simulink model "MLC_IPC_ctrl_r2018a"  (R2018a)
settings: Solver=ode4  StartTime=0.0  StopTime=Parameter.Time.TMax  FixedStep=Parameter.Time.dt  RelTol=1e-3  EnableMultiTasking=on
undefined symbols (not defined in the file or in its folder): Parameter, x2_t0
libraries: simulink x4
settings Model: Creator=Phoenix_Shao  LastModifiedBy=thisi
settings DataIOCC: MaxDataPoints=1000000  SaveFormat=Array  DSMLogging=off
settings OptimizationCC: ExpressionDepthLimit=2147483647  InitFltsAndDblsToZero=on  EfficientMapNaN2IntZero=off  LifeSpan=inf
settings DebuggingCC: SaveWithParameterizedLinksMsg=none  UnderspecifiedInitializationDetection=Classic  MergeDetectMultiDrivingBlocksExec=none  SignalResolutionControl=TryResolveAllWithWarning  SolverPrmCheckMsg=warning  MultiTaskDSMMsg=warning  MultiTaskCondExecSysMsg=none  FcnCallInpInsideContextMsg=warning  AllowSymbolicDim=off  StateNameClashWarn=warning  LibraryContextMissingDiagnostic=warning  SFUnexpectedBacktrackingDiag=warning  SFNoUnconditionalDefaultTransitionDiag=warning  SFExecutionAtInitializationDiag=none
settings HardwareCC: ProdBitPerPointer=32  ProdBitPerSizeT=32  ProdBitPerPtrDiffT=32  ProdLargestAtomicFloat=None  ProdIntDivRoundTo=Undefined  ProdEndianess=Unspecified  ProdWordSize=32  ProdHWDeviceType=32-bit Generic  TargetBitPerPointer=64  TargetBitPerSizeT=64  TargetBitPerPtrDiffT=64  TargetLongLongMode=on  TargetIntDivRoundTo=Zero  TargetEndianess=LittleEndian  TargetWordSize=64  TargetHWDeviceType=MATLAB Host  ProdEqTarget=off
settings ModelReferenceCC: PropagateSignalLabelsOutOfModel=off
settings ModelReferenceCC: ModelDependencies=|
  | MAP_x64.dll
  | OpenFAST-Simulink_x64.dll
  | FAST_SFunc.mexw64
settings SFSimCC: SimParseCustomCode=off
settings RTWCC: SystemTargetFile=accel.tlc  TemplateMakefile=accel_default_tmf  RTWVerbose=off
settings CodeAppCC: MaxIdLength=128  StateflowObjectComments=on
settings STFCustomTargetCC: GeneratePreprocessorConditionals=Disable all  MATLABClassNameForMDSCustomization=Simulink.SoftwareTarget.TargetSpecificTriggerConfigurationBase  SystemTargetFile=accel.tlc
settings ConfigComp: CovMetricSettings=dw  CovHtmlReporting=on  CovSaveCumulativeToWorkspaceVar=on  CovSaveSingleToWorkspaceVar=on  CovExternalEMLEnable=off

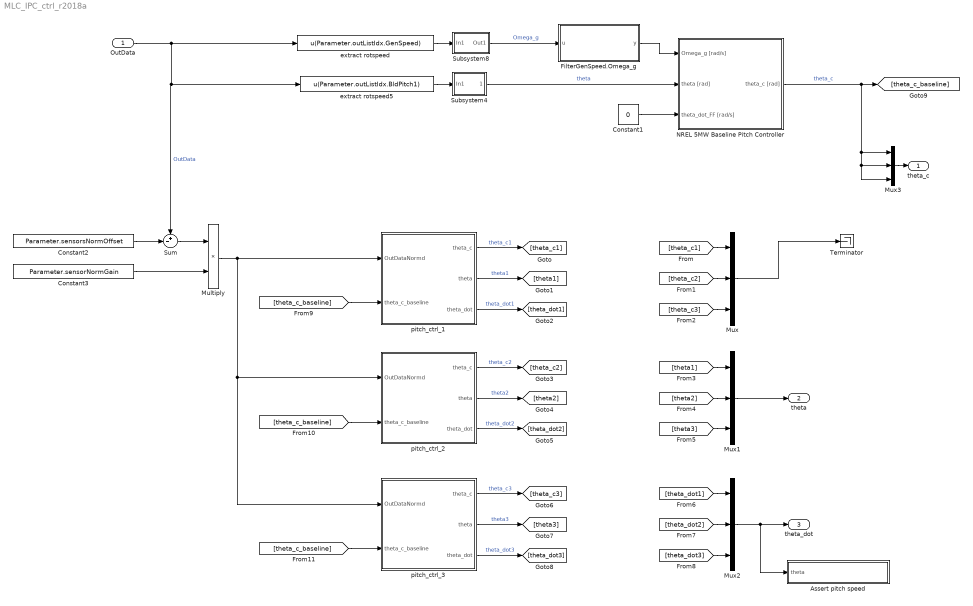
== system MLC_IPC_ctrl_r2018a ==
  OutData : Inport  PortDimensions=Parameter.MLC.totNSensors
  Assert pitch speed : Subsystem
  Constant1 : Constant  Value=0
  Constant2 : Constant  Value=Parameter.sensorsNormOffset
  Constant3 : Constant  Value=Parameter.sensorNormGain
  FilterGenSpeed.Omega_g : Subsystem
  Multiply : Product
  Mux{,1..3} (4 alike) : Mux  Inputs=3
  NREL 5MW Baseline Pitch Controller : Subsystem
  Subsystem4 : Subsystem
      mask Display: disp('deg2rad')
  Subsystem8 : Subsystem
      mask Display: disp('rpm2rad/s')
  Sum : Sum  Inputs=+-|
  Terminator : Terminator
  extract rotspeed : Fcn  Expr=u(Parameter.outListIdx.GenSpeed)
  extract rotspeed5 : Fcn  Expr=u(Parameter.outListIdx.BldPitch1)
  pitch_ctrl_1 : Subsystem
  pitch_ctrl_2 : Subsystem
  pitch_ctrl_3 : Subsystem
  "theta_c " : Outport  SignalName=theta_c
  theta : Outport  Port=2  SignalName=theta
  theta_dot : Outport  Port=3  SignalName=theta_dot
  wires:
  Mux/1 -> Terminator/1
  OutData/1 -> extract rotspeed5/1, Sum/1, extract rotspeed/1  "OutData"
  Mux1/1 -> theta/1
  Mux2/1 -> Assert pitch speed/1(theta), theta_dot/1
  FilterGenSpeed.Omega_g/1(y) -> NREL 5MW Baseline Pitch Controller/1(Omega_g [rad/s])
  Constant1/1 -> NREL 5MW Baseline Pitch Controller/3(theta_dot_FF [rad/s])
  Subsystem8/1(Out1) -> FilterGenSpeed.Omega_g/1(u)  "Omega_g"
  extract rotspeed/1 -> Subsystem8/1(In1)
  Subsystem4/1(Out1) -> NREL 5MW Baseline Pitch Controller/2(theta [rad])  "theta"
  extract rotspeed5/1 -> Subsystem4/1(In1)
  NREL 5MW Baseline Pitch Controller/1(theta_c [rad]) -> Mux3/1, Mux3/2, Mux3/3, [theta_c_baseline]  "theta_c"
  pitch_ctrl_1/1(theta_c) -> [theta_c1]  "theta_c1"
  pitch_ctrl_1/2(theta) -> [theta1]  "theta1"
  pitch_ctrl_1/3(theta_dot) -> [theta_dot1]  "theta_dot1"
  pitch_ctrl_2/1(theta_c) -> [theta_c2]  "theta_c2"
  pitch_ctrl_2/2(theta) -> [theta2]  "theta2"
  pitch_ctrl_2/3(theta_dot) -> [theta_dot2]  "theta_dot2"
  pitch_ctrl_3/1(theta_c) -> [theta_c3]  "theta_c3"
  pitch_ctrl_3/2(theta) -> [theta3]  "theta3"
  pitch_ctrl_3/3(theta_dot) -> [theta_dot3]  "theta_dot3"
  [theta_c1] -> Mux/1
  [theta_c2] -> Mux/2
  [theta_c3] -> Mux/3
  [theta1] -> Mux1/1
  [theta2] -> Mux1/2
  [theta3] -> Mux1/3
  [theta_dot1] -> Mux2/1
  [theta_dot2] -> Mux2/2
  [theta_dot3] -> Mux2/3
  [theta_c_baseline] -> pitch_ctrl_1/2(theta_c_baseline)
  [theta_c_baseline] -> pitch_ctrl_2/2(theta_c_baseline)
  [theta_c_baseline] -> pitch_ctrl_3/2(theta_c_baseline)
  Constant2/1 -> Sum/2
  Sum/1 -> Multiply/1
  Multiply/1 -> pitch_ctrl_3/1(OutDataNormd), pitch_ctrl_2/1(OutDataNormd), pitch_ctrl_1/1(OutDataNormd)
  Constant3/1 -> Multiply/2
  Mux3/1 -> "theta_c "/1

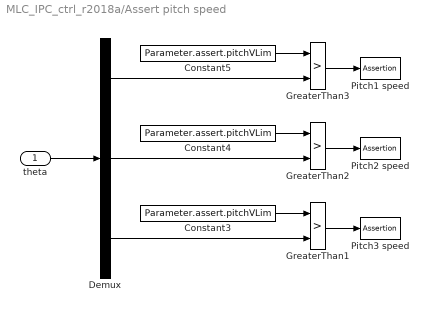
== system MLC_IPC_ctrl_r2018a/Assert pitch speed ==
  theta : Inport
  Constant3 : Constant  Value=Parameter.assert.pitchVLim
  Constant4 : Constant  Value=Parameter.assert.pitchVLim
  Constant5 : Constant  Value=Parameter.assert.pitchVLim
  Demux : Demux  Outputs=3
  GreaterThan1 : RelationalOperator  Operator=>  OutDataTypeStr=boolean  RndMeth=Simplest
  GreaterThan2 : RelationalOperator  Operator=>  OutDataTypeStr=boolean  RndMeth=Simplest
  GreaterThan3 : RelationalOperator  Operator=>  OutDataTypeStr=boolean  RndMeth=Simplest
  Pitch1 speed : Assertion
  Pitch2 speed : Assertion
  Pitch3 speed : Assertion
  wires:
  Constant5/1 -> GreaterThan3/1
  GreaterThan1/1 -> Pitch3 speed/1
  Constant3/1 -> GreaterThan1/1
  Constant4/1 -> GreaterThan2/1
  GreaterThan3/1 -> Pitch1 speed/1
  GreaterThan2/1 -> Pitch2 speed/1
  theta/1 -> Demux/1
  Demux/1 -> GreaterThan3/2
  Demux/2 -> GreaterThan2/2
  Demux/3 -> GreaterThan1/2

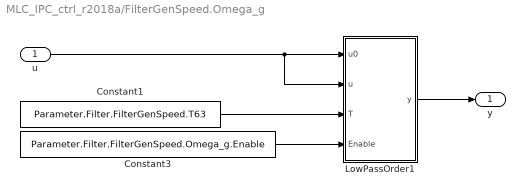
== system MLC_IPC_ctrl_r2018a/FilterGenSpeed.Omega_g ==
  u : Inport
  Constant1 : Constant  Value=Parameter.Filter.FilterGenSpeed.T63
  Constant3 : Constant  Value=Parameter.Filter.FilterGenSpeed.Omega_g.Enable
  LowPassOrder1 : Subsystem
  y : Outport
  wires:
  LowPassOrder1/1(y) -> y/1
  u/1 -> LowPassOrder1/2(u), LowPassOrder1/1(u0)
  Constant3/1 -> LowPassOrder1/4(Enable)
  Constant1/1 -> LowPassOrder1/3(T)

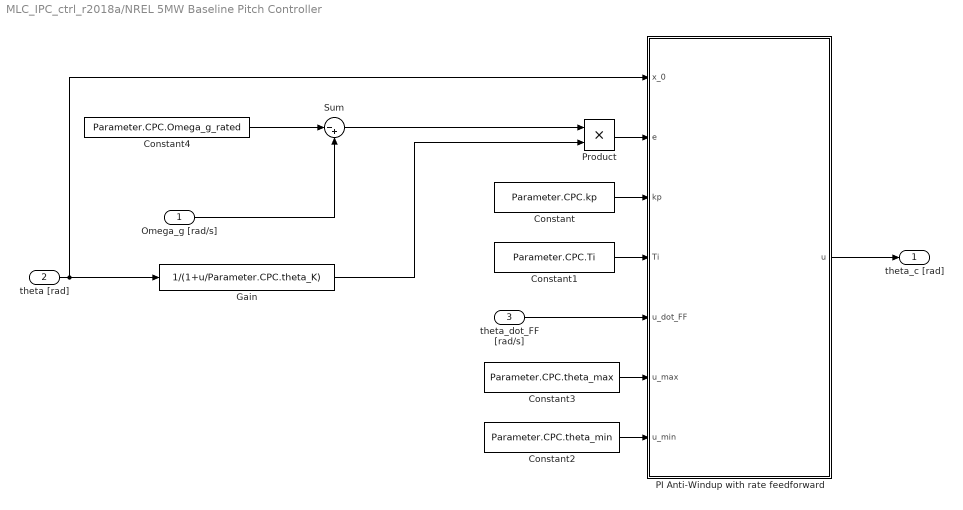
== system MLC_IPC_ctrl_r2018a/NREL 5MW Baseline Pitch Controller ==
  Omega_g [rad/s] : Inport
  theta [rad] : Inport  Port=2
  theta_dot_FF [rad/s] : Inport  Port=3
  Constant : Constant  Value=Parameter.CPC.kp
  Constant1 : Constant  Value=Parameter.CPC.Ti
  Constant2 : Constant  Value=Parameter.CPC.theta_min
  Constant3 : Constant  Value=Parameter.CPC.theta_max
  Constant4 : Constant  Value=Parameter.CPC.Omega_g_rated
  Gain : Fcn  Expr=1/(1+u/Parameter.CPC.theta_K)
  PI Anti-Windup with rate feedforward : Subsystem
  Product : Product  RndMeth=Zero
  Sum : Sum  Inputs=|-+
  theta_c [rad] : Outport
  wires:
  Constant4/1 -> Sum/1
  theta [rad]/1 -> Gain/1, PI Anti-Windup with rate feedforward/1(x_0)
  Omega_g [rad/s]/1 -> Sum/2
  Gain/1 -> Product/2
  Sum/1 -> Product/1
  Product/1 -> PI Anti-Windup with rate feedforward/2(e)
  theta_dot_FF [rad/s]/1 -> PI Anti-Windup with rate feedforward/5(u_dot_FF)
  PI Anti-Windup with rate feedforward/1(u) -> theta_c [rad]/1
  Constant/1 -> PI Anti-Windup with rate feedforward/3(kp)
  Constant1/1 -> PI Anti-Windup with rate feedforward/4(Ti)
  Constant2/1 -> PI Anti-Windup with rate feedforward/7(u_min)
  Constant3/1 -> PI Anti-Windup with rate feedforward/6(u_max)

== system MLC_IPC_ctrl_r2018a/Subsystem4 ==
  In1 : Inport
  deg in rad : Gain  Gain=2*pi/360  SaturateOnIntegerOverflow=on  OutDataTypeStr=Inherit: Same as input  ParamDataTypeStr=Inherit: Same as input
  Out1 : Outport
  wires:
  In1/1 -> deg in rad/1
  deg in rad/1 -> Out1/1

== system MLC_IPC_ctrl_r2018a/Subsystem8 ==
  In1 : Inport
  rpm in rad/s : Gain  Gain=2*pi/60  SaturateOnIntegerOverflow=on  OutDataTypeStr=Inherit: Same as input  ParamDataTypeStr=Inherit: Same as input
  Out1 : Outport
  wires:
  rpm in rad/s/1 -> Out1/1
  In1/1 -> rpm in rad/s/1

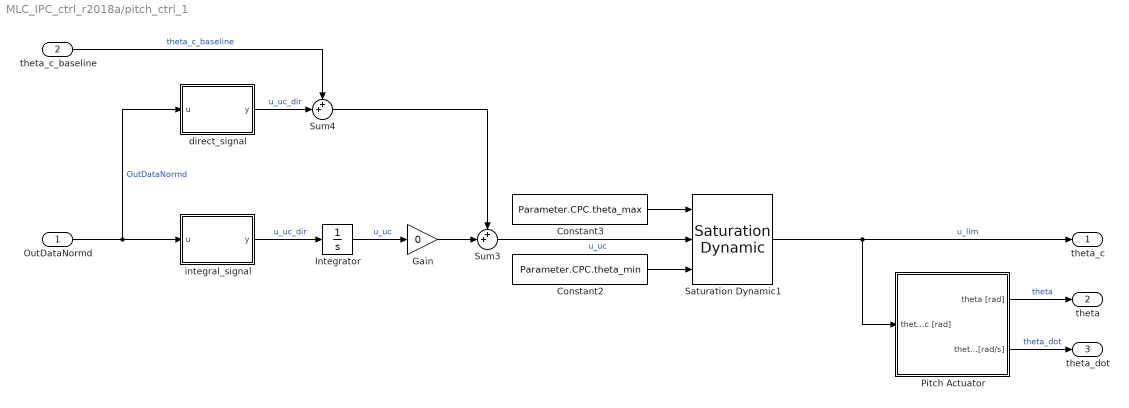
== system MLC_IPC_ctrl_r2018a/pitch_ctrl_1 ==
  OutDataNormd : Inport
  theta_c_baseline : Inport  Port=2
  Constant2 : Constant  Value=Parameter.CPC.theta_min
  Constant3 : Constant  Value=Parameter.CPC.theta_max
  Gain : Gain  Gain=0
  Integrator : Integrator  LimitOutput=on  UpperSaturationLimit=Parameter.CPC.theta_max  LowerSaturationLimit=Parameter.CPC.theta_min
  Pitch Actuator : Subsystem  AncestorBlock=Library/Models/Pitch Actuator
  Saturation Dynamic1 : simulink/Discontinuities/Saturation Dynamic  OutMin=[]  OutMax=[]  OutDataTypeStr=Inherit: Same as second input  OutDataType=fixdt(1, 16)  OutScaling=2^-10  DoSatur=off
  Sum3 : Sum  Inputs=++|
  Sum4 : Sum  Inputs=++|
  direct_signal : MATLAB Function  TreatAsAtomicUnit=on
  integral_signal : MATLAB Function  TreatAsAtomicUnit=on
  theta_c : Outport  PortDimensions=1
  theta : Outport  Port=2  PortDimensions=1
  theta_dot : Outport  Port=3  PortDimensions=1
  wires:
  OutDataNormd/1 -> integral_signal/1(u), direct_signal/1(u)  "OutDataNormd"
  Sum3/1 -> Saturation Dynamic1/2  "u_uc"
  Constant3/1 -> Saturation Dynamic1/1
  Constant2/1 -> Saturation Dynamic1/3
  Saturation Dynamic1/1 -> Pitch Actuator/1(theta_c [rad]), theta_c/1  "u_lim"
  Pitch Actuator/1(theta [rad]) -> theta/1  "theta"
  Pitch Actuator/2(theta_dot [rad/s]) -> theta_dot/1  "theta_dot"
  Integrator/1 -> Gain/1  "u_uc"
  theta_c_baseline/1 -> Sum4/1  "theta_c_baseline"
  direct_signal/1(y) -> Sum4/2  "u_uc_dir"
  Sum4/1 -> Sum3/1
  Gain/1 -> Sum3/2
  integral_signal/1(y) -> Integrator/1  "u_uc_dir"

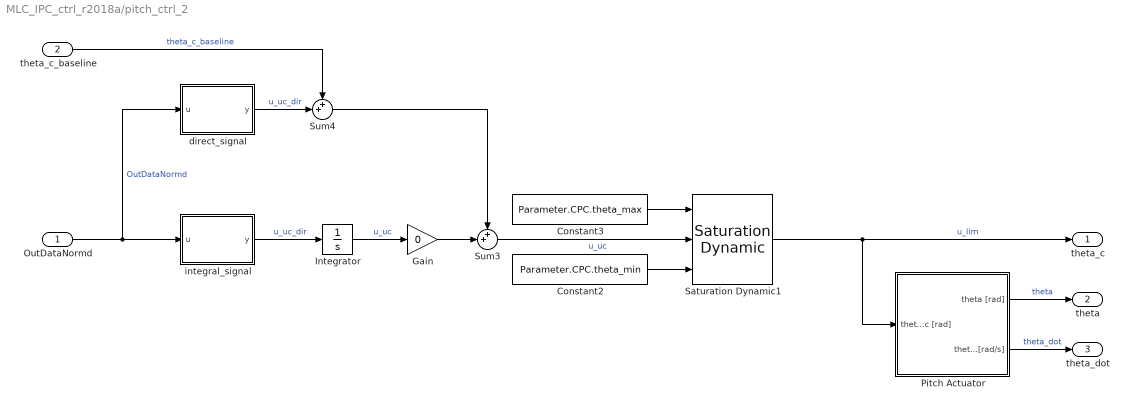
== system MLC_IPC_ctrl_r2018a/pitch_ctrl_2 ==
  OutDataNormd : Inport
  theta_c_baseline : Inport  Port=2
  Constant2 : Constant  Value=Parameter.CPC.theta_min
  Constant3 : Constant  Value=Parameter.CPC.theta_max
  Gain : Gain  Gain=0
  Integrator : Integrator  LimitOutput=on  UpperSaturationLimit=Parameter.CPC.theta_max  LowerSaturationLimit=Parameter.CPC.theta_min
  Pitch Actuator : Subsystem  AncestorBlock=Library/Models/Pitch Actuator
  Saturation Dynamic1 : simulink/Discontinuities/Saturation Dynamic  OutMin=[]  OutMax=[]  OutDataTypeStr=Inherit: Same as second input  OutDataType=fixdt(1, 16)  OutScaling=2^-10  DoSatur=off
  Sum3 : Sum  Inputs=++|
  Sum4 : Sum  Inputs=++|
  direct_signal : MATLAB Function  TreatAsAtomicUnit=on
  integral_signal : MATLAB Function  TreatAsAtomicUnit=on
  theta_c : Outport  PortDimensions=1
  theta : Outport  Port=2  PortDimensions=1
  theta_dot : Outport  Port=3  PortDimensions=1
  wires:
  integral_signal/1(y) -> Integrator/1  "u_uc_dir"
  Gain/1 -> Sum3/2
  Sum4/1 -> Sum3/1
  direct_signal/1(y) -> Sum4/2  "u_uc_dir"
  theta_c_baseline/1 -> Sum4/1  "theta_c_baseline"
  Integrator/1 -> Gain/1  "u_uc"
  Pitch Actuator/2(theta_dot [rad/s]) -> theta_dot/1  "theta_dot"
  Pitch Actuator/1(theta [rad]) -> theta/1  "theta"
  Saturation Dynamic1/1 -> theta_c/1, Pitch Actuator/1(theta_c [rad])  "u_lim"
  Constant2/1 -> Saturation Dynamic1/3
  Constant3/1 -> Saturation Dynamic1/1
  Sum3/1 -> Saturation Dynamic1/2  "u_uc"
  OutDataNormd/1 -> direct_signal/1(u), integral_signal/1(u)  "OutDataNormd"

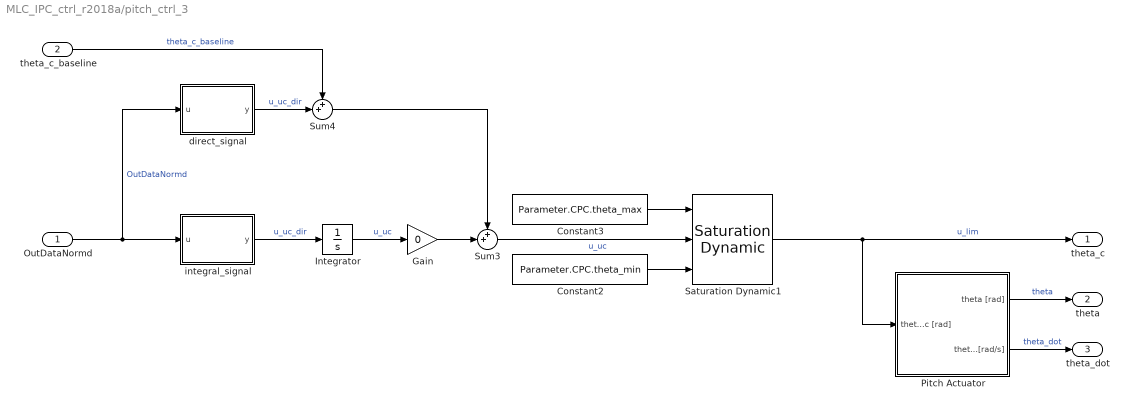
== system MLC_IPC_ctrl_r2018a/pitch_ctrl_3 ==
  OutDataNormd : Inport
  theta_c_baseline : Inport  Port=2
  Constant2 : Constant  Value=Parameter.CPC.theta_min
  Constant3 : Constant  Value=Parameter.CPC.theta_max
  Gain : Gain  Gain=0
  Integrator : Integrator  LimitOutput=on  UpperSaturationLimit=Parameter.CPC.theta_max  LowerSaturationLimit=Parameter.CPC.theta_min
  Pitch Actuator : Subsystem  AncestorBlock=Library/Models/Pitch Actuator
  Saturation Dynamic1 : simulink/Discontinuities/Saturation Dynamic  OutMin=[]  OutMax=[]  OutDataTypeStr=Inherit: Same as second input  OutDataType=fixdt(1, 16)  OutScaling=2^-10  DoSatur=off
  Sum3 : Sum  Inputs=++|
  Sum4 : Sum  Inputs=++|
  direct_signal : MATLAB Function  TreatAsAtomicUnit=on
  integral_signal : MATLAB Function  TreatAsAtomicUnit=on
  theta_c : Outport  PortDimensions=1
  theta : Outport  Port=2  PortDimensions=1
  theta_dot : Outport  Port=3  PortDimensions=1
  wires:
  OutDataNormd/1 -> integral_signal/1(u), direct_signal/1(u)  "OutDataNormd"
  Sum3/1 -> Saturation Dynamic1/2  "u_uc"
  Constant3/1 -> Saturation Dynamic1/1
  Constant2/1 -> Saturation Dynamic1/3
  Saturation Dynamic1/1 -> Pitch Actuator/1(theta_c [rad]), theta_c/1  "u_lim"
  Pitch Actuator/1(theta [rad]) -> theta/1  "theta"
  Pitch Actuator/2(theta_dot [rad/s]) -> theta_dot/1  "theta_dot"
  Integrator/1 -> Gain/1  "u_uc"
  theta_c_baseline/1 -> Sum4/1  "theta_c_baseline"
  direct_signal/1(y) -> Sum4/2  "u_uc_dir"
  Sum4/1 -> Sum3/1
  Gain/1 -> Sum3/2
  integral_signal/1(y) -> Integrator/1  "u_uc_dir"

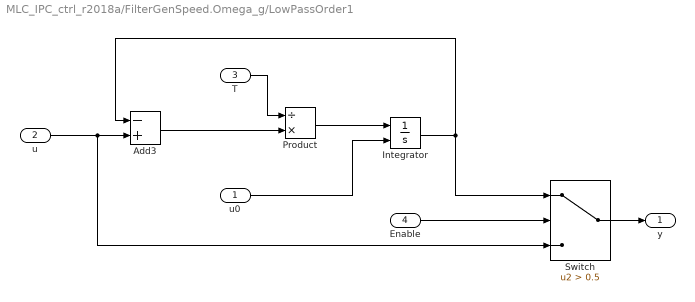
== system MLC_IPC_ctrl_r2018a/FilterGenSpeed.Omega_g/LowPassOrder1 ==
  u0 : Inport
  u : Inport  Port=2
  T : Inport  Port=3
  Enable : Inport  Port=4
  Add3 : Sum  Inputs=-+
  Integrator : Integrator  InitialConditionSource=external
  Product : Product  Inputs=/*  RndMeth=Zero
  Switch : Switch  Criteria=u2 > Threshold  Threshold=0.5
  y : Outport
  wires:
  u0/1 -> Integrator/2
  Switch/1 -> y/1
  Enable/1 -> Switch/2
  u/1 -> Add3/2, Switch/3
  T/1 -> Product/1
  Integrator/1 -> Add3/1, Switch/1
  Product/1 -> Integrator/1
  Add3/1 -> Product/2

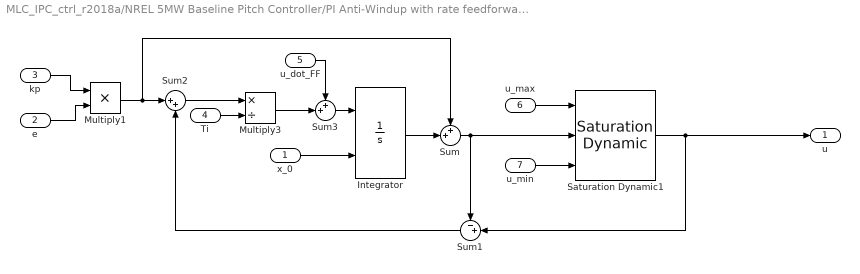
== system MLC_IPC_ctrl_r2018a/NREL 5MW Baseline Pitch Controller/PI Anti-Windup with rate feedforward ==
  x_0 : Inport
  e : Inport  Port=2
  kp : Inport  Port=3
  Ti : Inport  Port=4
  u_dot_FF : Inport  Port=5
  u_max : Inport  Port=6
  u_min : Inport  Port=7
  Integrator : Integrator  InitialConditionSource=external
  Multiply1 : Product  Inputs=**
  Multiply3 : Product  Inputs=*/
  Saturation Dynamic1 : simulink/Discontinuities/Saturation Dynamic  OutMin=[]  OutMax=[]  OutDataTypeStr=Inherit: Same as second input  OutDataType=fixdt(1, 16)  OutScaling=2^-10  DoSatur=off
  Sum : Sum  Inputs=++|
  Sum1 : Sum  Inputs=-+|
  Sum2 : Sum  Inputs=|++
  Sum3 : Sum  Inputs=++|
  u : Outport
  wires:
  Saturation Dynamic1/1 -> u/1, Sum1/2
  Integrator/1 -> Sum/2
  kp/1 -> Multiply1/1
  e/1 -> Multiply1/2
  Ti/1 -> Multiply3/2
  Multiply1/1 -> Sum/1, Sum2/1
  Sum2/1 -> Multiply3/1
  x_0/1 -> Integrator/2
  Multiply3/1 -> Sum3/2
  Sum3/1 -> Integrator/1
  u_dot_FF/1 -> Sum3/1
  u_min/1 -> Saturation Dynamic1/3
  Sum/1 -> Saturation Dynamic1/2, Sum1/1
  u_max/1 -> Saturation Dynamic1/1
  Sum1/1 -> Sum2/2

== system MLC_IPC_ctrl_r2018a/pitch_ctrl_1/Pitch Actuator ==
  theta_c [rad] : Inport
  Constant1 : Constant  Value=Parameter.IC.theta
  PT2 : Subsystem  mask{omega=Parameter.PitchActuator.omega, xi=Parameter.PitchActuator.xi, x1_max=Parameter.PitchActuator.theta_dot_max, x1_min=-Parameter.PitchActuator.theta_dot_max, x2_max=Parameter.PitchActuator.theta_max, x2_min=Parameter.PitchActuator.theta_min}
      mask prompts: omega "undamped natural frequency [rad/s]"; xi "damping factor [-]"; x1_max "Upper bound x1"; x1_min "Lower bound x1"; x2_max "Upper bound x2"; x2_min "Lower bound x2"
      mask Display:
      | disp(['omega = ',num2str(omega),'\n'...
      |     ,'xi = ',num2str(xi)])
      | port_label('output',1,'y')
      | port_label('output',2,'x1')
      | port_label('input',2,'y0')
      | port_label('input',1,'u')
  theta [rad] : Outport
  theta_dot [rad/s] : Outport  Port=2
  wires:
  Constant1/1 -> PT2/2(y0)
  theta_c [rad]/1 -> PT2/1(u)
  PT2/1(y) -> theta [rad]/1  "theta"
  PT2/2(x1) -> theta_dot [rad/s]/1  "theta_dot"

== system MLC_IPC_ctrl_r2018a/pitch_ctrl_2/Pitch Actuator ==
  theta_c [rad] : Inport
  Constant1 : Constant  Value=Parameter.IC.theta
  PT2 : Subsystem  mask{omega=Parameter.PitchActuator.omega, xi=Parameter.PitchActuator.xi, x1_max=Parameter.PitchActuator.theta_dot_max, x1_min=-Parameter.PitchActuator.theta_dot_max, x2_max=Parameter.PitchActuator.theta_max, x2_min=Parameter.PitchActuator.theta_min}
      mask prompts: omega "undamped natural frequency [rad/s]"; xi "damping factor [-]"; x1_max "Upper bound x1"; x1_min "Lower bound x1"; x2_max "Upper bound x2"; x2_min "Lower bound x2"
      mask Display:
      | disp(['omega = ',num2str(omega),'\n'...
      |     ,'xi = ',num2str(xi)])
      | port_label('output',1,'y')
      | port_label('output',2,'x1')
      | port_label('input',2,'y0')
      | port_label('input',1,'u')
  theta [rad] : Outport
  theta_dot [rad/s] : Outport  Port=2
  wires:
  PT2/2(x1) -> theta_dot [rad/s]/1  "theta_dot"
  PT2/1(y) -> theta [rad]/1  "theta"
  theta_c [rad]/1 -> PT2/1(u)
  Constant1/1 -> PT2/2(y0)

== system MLC_IPC_ctrl_r2018a/pitch_ctrl_3/Pitch Actuator ==
  theta_c [rad] : Inport
  Constant1 : Constant  Value=Parameter.IC.theta
  PT2 : Subsystem  mask{omega=Parameter.PitchActuator.omega, xi=Parameter.PitchActuator.xi, x1_max=Parameter.PitchActuator.theta_dot_max, x1_min=-Parameter.PitchActuator.theta_dot_max, x2_max=Parameter.PitchActuator.theta_max, x2_min=Parameter.PitchActuator.theta_min}
      mask prompts: omega "undamped natural frequency [rad/s]"; xi "damping factor [-]"; x1_max "Upper bound x1"; x1_min "Lower bound x1"; x2_max "Upper bound x2"; x2_min "Lower bound x2"
      mask Display:
      | disp(['omega = ',num2str(omega),'\n'...
      |     ,'xi = ',num2str(xi)])
      | port_label('output',1,'y')
      | port_label('output',2,'x1')
      | port_label('input',2,'y0')
      | port_label('input',1,'u')
  theta [rad] : Outport
  theta_dot [rad/s] : Outport  Port=2
  wires:
  Constant1/1 -> PT2/2(y0)
  theta_c [rad]/1 -> PT2/1(u)
  PT2/1(y) -> theta [rad]/1  "theta"
  PT2/2(x1) -> theta_dot [rad/s]/1  "theta_dot"

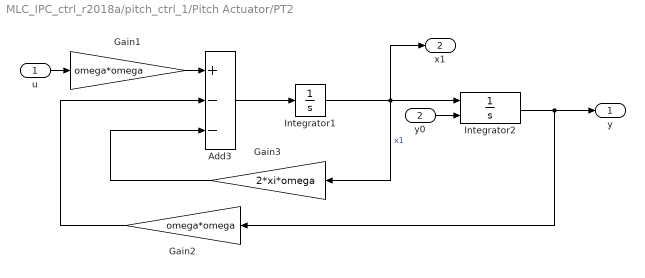
== system MLC_IPC_ctrl_r2018a/pitch_ctrl_1/Pitch Actuator/PT2 ==
  u : Inport
  y0 : Inport  Port=2
  Add3 : Sum  Inputs=+--
  Gain1 : Gain  Gain=omega*omega  SaturateOnIntegerOverflow=on  OutDataTypeStr=Inherit: Same as input  ParamDataTypeStr=Inherit: Same as input
  Gain2 : Gain  Gain=omega*omega  SaturateOnIntegerOverflow=on  OutDataTypeStr=Inherit: Same as input  ParamDataTypeStr=Inherit: Same as input
  Gain3 : Gain  Gain=2*xi*omega  SaturateOnIntegerOverflow=on  OutDataTypeStr=Inherit: Same as input  ParamDataTypeStr=Inherit: Same as input
  Integrator1 : Integrator  LimitOutput=on  UpperSaturationLimit=x1_max  LowerSaturationLimit=x1_min
  Integrator2 : Integrator  InitialConditionSource=external  InitialCondition=x2_t0  LimitOutput=on  UpperSaturationLimit=x2_max  LowerSaturationLimit=x2_min
  y : Outport
  x1 : Outport  Port=2
  wires:
  Integrator2/1 -> y/1, Gain2/1
  y0/1 -> Integrator2/2
  Integrator1/1 -> Integrator2/1, Gain3/1, x1/1  "x1"
  Gain2/1 -> Add3/2
  Gain1/1 -> Add3/1
  Add3/1 -> Integrator1/1
  u/1 -> Gain1/1
  Gain3/1 -> Add3/3

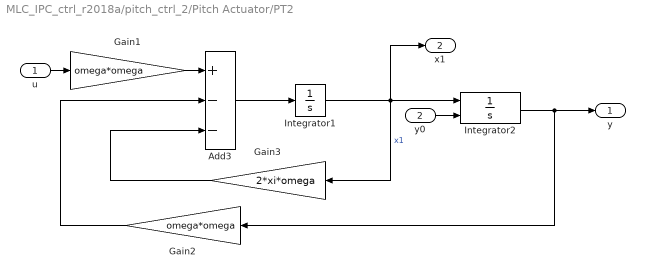
== system MLC_IPC_ctrl_r2018a/pitch_ctrl_2/Pitch Actuator/PT2 ==
  u : Inport
  y0 : Inport  Port=2
  Add3 : Sum  Inputs=+--
  Gain1 : Gain  Gain=omega*omega  SaturateOnIntegerOverflow=on  OutDataTypeStr=Inherit: Same as input  ParamDataTypeStr=Inherit: Same as input
  Gain2 : Gain  Gain=omega*omega  SaturateOnIntegerOverflow=on  OutDataTypeStr=Inherit: Same as input  ParamDataTypeStr=Inherit: Same as input
  Gain3 : Gain  Gain=2*xi*omega  SaturateOnIntegerOverflow=on  OutDataTypeStr=Inherit: Same as input  ParamDataTypeStr=Inherit: Same as input
  Integrator1 : Integrator  LimitOutput=on  UpperSaturationLimit=x1_max  LowerSaturationLimit=x1_min
  Integrator2 : Integrator  InitialConditionSource=external  InitialCondition=x2_t0  LimitOutput=on  UpperSaturationLimit=x2_max  LowerSaturationLimit=x2_min
  y : Outport
  x1 : Outport  Port=2
  wires:
  Gain3/1 -> Add3/3
  u/1 -> Gain1/1
  Add3/1 -> Integrator1/1
  Gain1/1 -> Add3/1
  Gain2/1 -> Add3/2
  Integrator1/1 -> x1/1, Gain3/1, Integrator2/1  "x1"
  y0/1 -> Integrator2/2
  Integrator2/1 -> Gain2/1, y/1

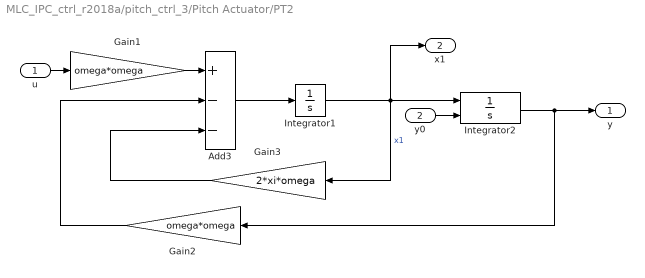
== system MLC_IPC_ctrl_r2018a/pitch_ctrl_3/Pitch Actuator/PT2 ==
  u : Inport
  y0 : Inport  Port=2
  Add3 : Sum  Inputs=+--
  Gain1 : Gain  Gain=omega*omega  SaturateOnIntegerOverflow=on  OutDataTypeStr=Inherit: Same as input  ParamDataTypeStr=Inherit: Same as input
  Gain2 : Gain  Gain=omega*omega  SaturateOnIntegerOverflow=on  OutDataTypeStr=Inherit: Same as input  ParamDataTypeStr=Inherit: Same as input
  Gain3 : Gain  Gain=2*xi*omega  SaturateOnIntegerOverflow=on  OutDataTypeStr=Inherit: Same as input  ParamDataTypeStr=Inherit: Same as input
  Integrator1 : Integrator  LimitOutput=on  UpperSaturationLimit=x1_max  LowerSaturationLimit=x1_min
  Integrator2 : Integrator  InitialConditionSource=external  InitialCondition=x2_t0  LimitOutput=on  UpperSaturationLimit=x2_max  LowerSaturationLimit=x2_min
  y : Outport
  x1 : Outport  Port=2
  wires:
  Integrator2/1 -> y/1, Gain2/1
  y0/1 -> Integrator2/2
  Integrator1/1 -> Integrator2/1, Gain3/1, x1/1  "x1"
  Gain2/1 -> Add3/2
  Gain1/1 -> Add3/1
  Add3/1 -> Integrator1/1
  u/1 -> Gain1/1
  Gain3/1 -> Add3/3

== matlab function MLC_IPC_ctrl_r2018a/pitch_ctrl_1/integral_signal ==
  data: u input; y output
function y = fcn(u)
y = sin((-9.576));

== matlab function MLC_IPC_ctrl_r2018a/pitch_ctrl_1/direct_signal ==
  data: u input; y output
function y = fcn(u)
y = ((-2.784) + (-6.435));

== matlab function MLC_IPC_ctrl_r2018a/pitch_ctrl_2/direct_signal ==
  data: u input; y output
function y = fcn(u)
y = sin((-9.576));

== matlab function MLC_IPC_ctrl_r2018a/pitch_ctrl_2/integral_signal ==
  data: u input; y output
function y = fcn(u)
y = (u(5) * 8.753);

== matlab function MLC_IPC_ctrl_r2018a/pitch_ctrl_3/direct_signal ==
  data: u input; y output
function y = fcn(u)
y = (my_div(u(2),u(74)));

== matlab function MLC_IPC_ctrl_r2018a/pitch_ctrl_3/integral_signal ==
  data: u input; y output
function y = fcn(u)
y = tanh((-6.19));
